simulink model "koen_observer_pll_model_annotated"  (R2024b)
settings: Solver=FixedStepDiscrete  StartTime=0.0  StopTime=0.05  FixedStep=6.25e-05  RelTol=1e-3
PreLoadFcn:
  | FOC_TS_SEC=6.25e-05; FOC_RS_OHM=0.53; FOC_LS_H=0.0006; FOC_FLUX_WB=0.0078; FOC_FLUX_LIMIT_RATIO=1.5; FOC_OBS_PLL_KP=180; FOC_OBS_PLL_KI=6000; FOC_OBS_PLL_INTEGRAL_LIMIT=700; FOC_OBS_SPEED_LIMIT_RAD_S=1200; FOC_OBS_SPEED_FILTER_ALPHA=0.2; FOC_OBS_THETA_COMP_RAD=2.7239; FOC_TWO_PI=6.283185307179586;
settings Model: Creator=10095  LastModifiedBy=10095

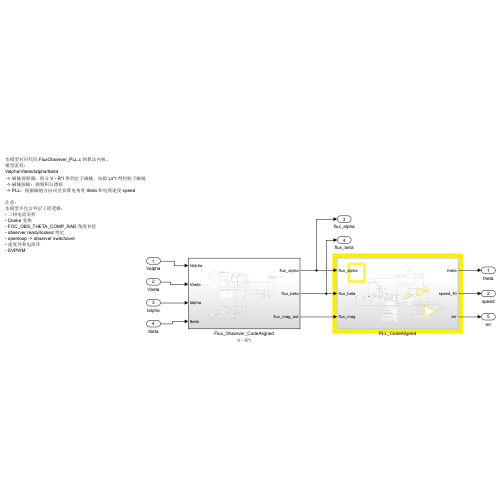
[thumbnail: Simulink's stored preview of the top-level diagram]
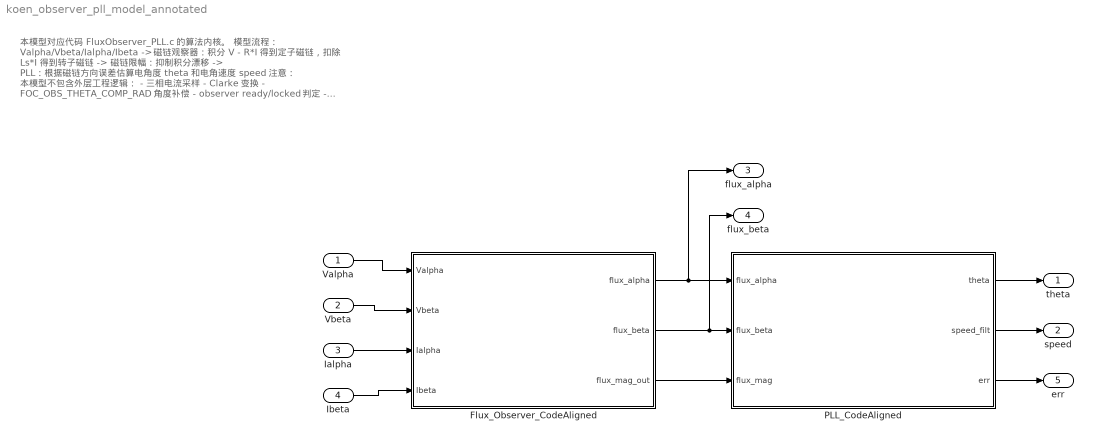
== system koen_observer_pll_model_annotated ==
  note: 本模型对应代码 FluxObserver_PLL.c 的算法内核。
      | 模型流程：
      | Valpha/Vbeta/Ialpha/Ibeta
      |  -> 磁链观察器：积分 V - R*I 得到定子磁链，扣除 Ls*I 得到转子磁链
      |  -> 磁链限幅：抑制积分漂移
      |  -> PLL：根据磁链方向误差估算电角度 theta 和电角速度 speed
      |
      | 注意：
      | 本模型不包含外层工程逻辑：
      | - 三相电流采样
      | - Clarke 变换
      | - FOC_OBS_THETA_COMP_RAD 角度补偿
      | - observer ready/locked 判定
      | - openloop -> observer switchover
      | - 速度环和电流环
      | - SVPWM
  Valpha : Inport
  Vbeta : Inport  Port=2
  Ialpha : Inport  Port=3
  Ibeta : Inport  Port=4
  Flux_Observer_CodeAligned : Subsystem  Description=|
      | Flux_Observer_CodeAligned：按 FluxObserver_PLL.c 更新定子磁链、扣除 Ls*i，并加入磁链幅值限幅。
      | 
      | 【代码对齐补充注释】
      | 定子磁链变化率计算模块。\n根据电机电压方程：psi_s_alpha_dot = Valpha - Rs*Ialpha。\nbeta 轴同理：psi_s_beta_dot = Vbeta - Rs*Ibeta。\n对应 FluxObserver_PLL.c 中 Ts * (ualpha - Rs*ialpha) 里的括号部分。
      settings: AttributesFormatString=V - R*I
  PLL_CodeAligned : Subsystem  Description=PLL_CodeAligned：按 FluxObserver_PLL.c 计算归一化相位误差、积分限幅、速度限幅、速度滤波和 theta wrap。
  theta : Outport
  speed : Outport  Port=2
  flux_alpha : Outport  Port=3
  flux_beta : Outport  Port=4
  err : Outport  Port=5
  wires:
  Valpha/1 -> Flux_Observer_CodeAligned/1(Valpha)
  Ialpha/1 -> Flux_Observer_CodeAligned/3(Ialpha)
  Vbeta/1 -> Flux_Observer_CodeAligned/2(Vbeta)
  Ibeta/1 -> Flux_Observer_CodeAligned/4(Ibeta)
  PLL_CodeAligned/1(theta) -> theta/1
  Flux_Observer_CodeAligned/3(flux_mag_out) -> PLL_CodeAligned/3(flux_mag)
  Flux_Observer_CodeAligned/2(flux_beta) -> PLL_CodeAligned/2(flux_beta), flux_beta/1
  PLL_CodeAligned/3(err) -> err/1
  Flux_Observer_CodeAligned/1(flux_alpha) -> flux_alpha/1, PLL_CodeAligned/1(flux_alpha)
  PLL_CodeAligned/2(speed_filt) -> speed/1

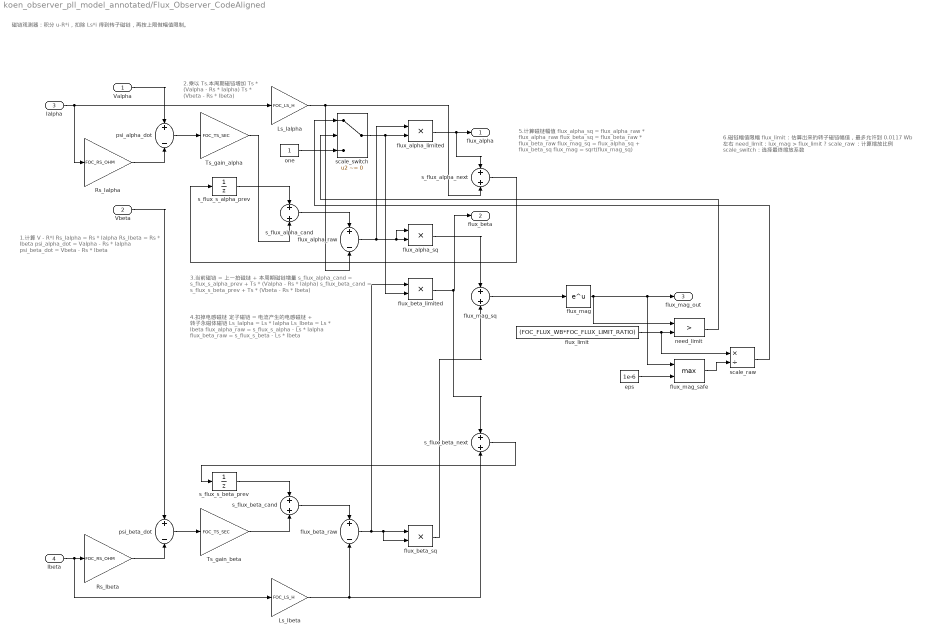
== system koen_observer_pll_model_annotated/Flux_Observer_CodeAligned ==
  note: 6.磁链幅值限幅
      | flux_limit：估算出来的转子磁链幅值，最多允许到 0.0117 Wb 左右
      | need_limit：lux_mag > flux_limit ?
      | scale_raw：计算缩放比例
      | scale_switch：选择最终缩放系数
  note: 5.计算磁链幅值
      | flux_alpha_sq = flux_alpha_raw * flux_alpha_raw
      | flux_beta_sq  = flux_beta_raw  * flux_beta_raw
      | flux_mag_sq   = flux_alpha_sq + flux_beta_sq
      | flux_mag      = sqrt(flux_mag_sq)
  note: 4.扣掉电感磁链
      | 定子磁链 = 电流产生的电感磁链 + 转子永磁体磁链
      | Ls_Ialpha = Ls * Ialpha
      | Ls_Ibeta  = Ls * Ibeta
      |
      | flux_alpha_raw = s_flux_s_alpha - Ls * Ialpha
      | flux_beta_raw  = s_flux_s_beta  - Ls * Ibeta
  note: 3.当前磁链 = 上一拍磁链 + 本周期磁链增量
      | s_flux_alpha_cand = s_flux_s_alpha_prev + Ts * (Valpha - Rs * Ialpha)
      | s_flux_beta_cand = s_flux_s_beta_prev + Ts * (Vbeta - Rs * Ibeta)
  note: 2.乘以 Ts.本周期磁链增加
      | Ts * (Valpha - Rs * Ialpha)
      | Ts * (Vbeta - Rs * Ibeta)
  note: 1.计算 V - R*I
      | Rs_Ialpha = Rs * Ialpha
      | Rs_Ibeta = Rs * Ibeta
      |
      | psi_alpha_dot = Valpha - Rs * Ialpha
      | psi_beta_dot = Vbeta - Rs * Ibeta
  note: 磁链观测器：积分 u-R*i，扣除 Ls*i 得到转子磁链，再按上限做幅值限制。
  Valpha : Inport  Description=|
      | 【代码对齐补充注释】
      | 输入端口：控制器输出的 alpha/beta 电压。\nValpha/Vbeta 对应代码 FluxObserver_PLL_t 中的 Valpha_I、Vbeta_I。\n这些电压是磁链积分的输入，来自电流环最终输出的 alpha/beta 电压。
      settings: AttributesFormatString=V - R*I
  Vbeta : Inport  Description=|  Port=2
      | 【代码对齐补充注释】
      | 输入端口：控制器输出的 alpha/beta 电压。\nValpha/Vbeta 对应代码 FluxObserver_PLL_t 中的 Valpha_I、Vbeta_I。\n这些电压是磁链积分的输入，来自电流环最终输出的 alpha/beta 电压。
      settings: AttributesFormatString=V - R*I
  Ialpha : Inport  Description=|  Port=3
      | 【代码对齐补充注释】
      | 输入端口：三相电流经过 Clarke 变换后的 alpha/beta 电流。\nIalpha/Ibeta 对应代码 FluxObserver_PLL_t 中的 Ialpha_I、Ibeta_I。\n这些电流用于计算 Rs*I 压降和 Ls*I 电感磁链。
      settings: AttributesFormatString=V - R*I
  Ibeta : Inport  Description=|  Port=4
      | 【代码对齐补充注释】
      | 输入端口：三相电流经过 Clarke 变换后的 alpha/beta 电流。\nIalpha/Ibeta 对应代码 FluxObserver_PLL_t 中的 Ialpha_I、Ibeta_I。\n这些电流用于计算 Rs*I 压降和 Ls*I 电感磁链。
      settings: AttributesFormatString=V - R*I
  Ls_Ialpha : Gain  Description=|  Gain=FOC_LS_H
      | 【代码对齐补充注释】
      | 输入端口：三相电流经过 Clarke 变换后的 alpha/beta 电流。\nIalpha/Ibeta 对应代码 FluxObserver_PLL_t 中的 Ialpha_I、Ibeta_I。\n这些电流用于计算 Rs*I 压降和 Ls*I 电感磁链。
      settings: AttributesFormatString=Ls * I
  Ls_Ibeta : Gain  Description=|  Gain=FOC_LS_H
      | 【代码对齐补充注释】
      | 输入端口：三相电流经过 Clarke 变换后的 alpha/beta 电流。\nIalpha/Ibeta 对应代码 FluxObserver_PLL_t 中的 Ialpha_I、Ibeta_I。\n这些电流用于计算 Rs*I 压降和 Ls*I 电感磁链。
      settings: AttributesFormatString=Ls * I
  Rs_Ialpha : Gain  Description=|  Gain=FOC_RS_OHM
      | 【代码对齐补充注释】
      | 输入端口：三相电流经过 Clarke 变换后的 alpha/beta 电流。\nIalpha/Ibeta 对应代码 FluxObserver_PLL_t 中的 Ialpha_I、Ibeta_I。\n这些电流用于计算 Rs*I 压降和 Ls*I 电感磁链。
      settings: AttributesFormatString=V - R*I
  Rs_Ibeta : Gain  Description=|  Gain=FOC_RS_OHM
      | 【代码对齐补充注释】
      | 输入端口：三相电流经过 Clarke 变换后的 alpha/beta 电流。\nIalpha/Ibeta 对应代码 FluxObserver_PLL_t 中的 Ialpha_I、Ibeta_I。\n这些电流用于计算 Rs*I 压降和 Ls*I 电感磁链。
      settings: AttributesFormatString=V - R*I
  Ts_gain_alpha : Gain  Description=|  Gain=FOC_TS_SEC
      | 【代码对齐补充注释】
      | 定子磁链变化率计算模块。\n根据电机电压方程：psi_s_alpha_dot = Valpha - Rs*Ialpha。\nbeta 轴同理：psi_s_beta_dot = Vbeta - Rs*Ibeta。\n对应 FluxObserver_PLL.c 中 Ts * (ualpha - Rs*ialpha) 里的括号部分。
      settings: AttributesFormatString=Ts * ψdot
  Ts_gain_beta : Gain  Description=|  Gain=FOC_TS_SEC
      | 【代码对齐补充注释】
      | 定子磁链变化率计算模块。\n根据电机电压方程：psi_s_alpha_dot = Valpha - Rs*Ialpha。\nbeta 轴同理：psi_s_beta_dot = Vbeta - Rs*Ibeta。\n对应 FluxObserver_PLL.c 中 Ts * (ualpha - Rs*ialpha) 里的括号部分。
      settings: AttributesFormatString=Ts * ψdot
  eps : Constant  Description=|  Value=1e-6
      | 【代码对齐补充注释】
      | 定子磁链变化率计算模块。\n根据电机电压方程：psi_s_alpha_dot = Valpha - Rs*Ialpha。\nbeta 轴同理：psi_s_beta_dot = Vbeta - Rs*Ibeta。\n对应 FluxObserver_PLL.c 中 Ts * (ualpha - Rs*ialpha) 里的括号部分。
      settings: AttributesFormatString=V - R*I
  flux_alpha_limited : Product  Description=|
      | 【代码对齐补充注释】
      | 定子磁链变化率计算模块。\n根据电机电压方程：psi_s_alpha_dot = Valpha - Rs*Ialpha。\nbeta 轴同理：psi_s_beta_dot = Vbeta - Rs*Ibeta。\n对应 FluxObserver_PLL.c 中 Ts * (ualpha - Rs*ialpha) 里的括号部分。
      settings: AttributesFormatString=limit |ψr|
  flux_alpha_raw : Sum  Description=|  Inputs=+-
      | 【代码对齐补充注释】
      | 定子磁链变化率计算模块。\n根据电机电压方程：psi_s_alpha_dot = Valpha - Rs*Ialpha。\nbeta 轴同理：psi_s_beta_dot = Vbeta - Rs*Ibeta。\n对应 FluxObserver_PLL.c 中 Ts * (ualpha - Rs*ialpha) 里的括号部分。
      settings: AttributesFormatString=ψr = ψs - LsI
  flux_alpha_sq : Product  Description=|
      | 【代码对齐补充注释】
      | 定子磁链变化率计算模块。\n根据电机电压方程：psi_s_alpha_dot = Valpha - Rs*Ialpha。\nbeta 轴同理：psi_s_beta_dot = Vbeta - Rs*Ibeta。\n对应 FluxObserver_PLL.c 中 Ts * (ualpha - Rs*ialpha) 里的括号部分。
      settings: AttributesFormatString=V - R*I
  flux_beta_limited : Product  Description=|
      | 【代码对齐补充注释】
      | 定子磁链变化率计算模块。\n根据电机电压方程：psi_s_alpha_dot = Valpha - Rs*Ialpha。\nbeta 轴同理：psi_s_beta_dot = Vbeta - Rs*Ibeta。\n对应 FluxObserver_PLL.c 中 Ts * (ualpha - Rs*ialpha) 里的括号部分。
      settings: AttributesFormatString=limit |ψr|
  flux_beta_raw : Sum  Description=|  Inputs=+-
      | 【代码对齐补充注释】
      | 定子磁链变化率计算模块。\n根据电机电压方程：psi_s_alpha_dot = Valpha - Rs*Ialpha。\nbeta 轴同理：psi_s_beta_dot = Vbeta - Rs*Ibeta。\n对应 FluxObserver_PLL.c 中 Ts * (ualpha - Rs*ialpha) 里的括号部分。
      settings: AttributesFormatString=ψr = ψs - LsI
  flux_beta_sq : Product  Description=|
      | 【代码对齐补充注释】
      | 定子磁链变化率计算模块。\n根据电机电压方程：psi_s_alpha_dot = Valpha - Rs*Ialpha。\nbeta 轴同理：psi_s_beta_dot = Vbeta - Rs*Ibeta。\n对应 FluxObserver_PLL.c 中 Ts * (ualpha - Rs*ialpha) 里的括号部分。
      settings: AttributesFormatString=V - R*I
  flux_limit : Constant  Description=|  Value=(FOC_FLUX_WB*FOC_FLUX_LIMIT_RATIO)
      | 【代码对齐补充注释】
      | 定子磁链变化率计算模块。\n根据电机电压方程：psi_s_alpha_dot = Valpha - Rs*Ialpha。\nbeta 轴同理：psi_s_beta_dot = Vbeta - Rs*Ibeta。\n对应 FluxObserver_PLL.c 中 Ts * (ualpha - Rs*ialpha) 里的括号部分。
      settings: AttributesFormatString=limit |ψr|
  flux_mag : Math  Description=|
      | 【代码对齐补充注释】
      | 定子磁链变化率计算模块。\n根据电机电压方程：psi_s_alpha_dot = Valpha - Rs*Ialpha。\nbeta 轴同理：psi_s_beta_dot = Vbeta - Rs*Ibeta。\n对应 FluxObserver_PLL.c 中 Ts * (ualpha - Rs*ialpha) 里的括号部分。
      settings: AttributesFormatString=|ψr|
  flux_mag_safe : MinMax  Description=|  Function=max  Inputs=2
      | 【代码对齐补充注释】
      | 定子磁链变化率计算模块。\n根据电机电压方程：psi_s_alpha_dot = Valpha - Rs*Ialpha。\nbeta 轴同理：psi_s_beta_dot = Vbeta - Rs*Ibeta。\n对应 FluxObserver_PLL.c 中 Ts * (ualpha - Rs*ialpha) 里的括号部分。
      settings: AttributesFormatString=|ψr|
  flux_mag_sq : Sum  Description=|
      | 【代码对齐补充注释】
      | 定子磁链变化率计算模块。\n根据电机电压方程：psi_s_alpha_dot = Valpha - Rs*Ialpha。\nbeta 轴同理：psi_s_beta_dot = Vbeta - Rs*Ibeta。\n对应 FluxObserver_PLL.c 中 Ts * (ualpha - Rs*ialpha) 里的括号部分。
      settings: AttributesFormatString=|ψr|
  need_limit : RelationalOperator  Description=|  Operator=>  OutDataTypeStr=boolean  RndMeth=Simplest  InputSameDT=off
      | 【代码对齐补充注释】
      | 定子磁链变化率计算模块。\n根据电机电压方程：psi_s_alpha_dot = Valpha - Rs*Ialpha。\nbeta 轴同理：psi_s_beta_dot = Vbeta - Rs*Ibeta。\n对应 FluxObserver_PLL.c 中 Ts * (ualpha - Rs*ialpha) 里的括号部分。
      settings: AttributesFormatString=limit |ψr|
  one : Constant  Description=|
      | 【代码对齐补充注释】
      | 定子磁链变化率计算模块。\n根据电机电压方程：psi_s_alpha_dot = Valpha - Rs*Ialpha。\nbeta 轴同理：psi_s_beta_dot = Vbeta - Rs*Ibeta。\n对应 FluxObserver_PLL.c 中 Ts * (ualpha - Rs*ialpha) 里的括号部分。
      settings: AttributesFormatString=V - R*I
  psi_alpha_dot : Sum  Description=|  Inputs=+-
      | 【代码对齐补充注释】
      | 定子磁链变化率计算模块。\n根据电机电压方程：psi_s_alpha_dot = Valpha - Rs*Ialpha。\nbeta 轴同理：psi_s_beta_dot = Vbeta - Rs*Ibeta。\n对应 FluxObserver_PLL.c 中 Ts * (ualpha - Rs*ialpha) 里的括号部分。
      settings: AttributesFormatString=V - R*I
  psi_beta_dot : Sum  Description=|  Inputs=+-
      | 【代码对齐补充注释】
      | 定子磁链变化率计算模块。\n根据电机电压方程：psi_s_alpha_dot = Valpha - Rs*Ialpha。\nbeta 轴同理：psi_s_beta_dot = Vbeta - Rs*Ibeta。\n对应 FluxObserver_PLL.c 中 Ts * (ualpha - Rs*ialpha) 里的括号部分。
      settings: AttributesFormatString=V - R*I
  s_flux_alpha_cand : Sum  Description=|
      | 【代码对齐补充注释】
      | 定子磁链变化率计算模块。\n根据电机电压方程：psi_s_alpha_dot = Valpha - Rs*Ialpha。\nbeta 轴同理：psi_s_beta_dot = Vbeta - Rs*Ibeta。\n对应 FluxObserver_PLL.c 中 Ts * (ualpha - Rs*ialpha) 里的括号部分。
      settings: AttributesFormatString=V - R*I
  s_flux_alpha_next : Sum  Description=|
      | 【代码对齐补充注释】
      | 定子磁链变化率计算模块。\n根据电机电压方程：psi_s_alpha_dot = Valpha - Rs*Ialpha。\nbeta 轴同理：psi_s_beta_dot = Vbeta - Rs*Ibeta。\n对应 FluxObserver_PLL.c 中 Ts * (ualpha - Rs*ialpha) 里的括号部分。
      settings: AttributesFormatString=V - R*I
  s_flux_beta_cand : Sum  Description=|
      | 【代码对齐补充注释】
      | 定子磁链变化率计算模块。\n根据电机电压方程：psi_s_alpha_dot = Valpha - Rs*Ialpha。\nbeta 轴同理：psi_s_beta_dot = Vbeta - Rs*Ibeta。\n对应 FluxObserver_PLL.c 中 Ts * (ualpha - Rs*ialpha) 里的括号部分。
      settings: AttributesFormatString=V - R*I
  s_flux_beta_next : Sum  Description=|
      | 【代码对齐补充注释】
      | 定子磁链变化率计算模块。\n根据电机电压方程：psi_s_alpha_dot = Valpha - Rs*Ialpha。\nbeta 轴同理：psi_s_beta_dot = Vbeta - Rs*Ibeta。\n对应 FluxObserver_PLL.c 中 Ts * (ualpha - Rs*ialpha) 里的括号部分。
      settings: AttributesFormatString=V - R*I
  s_flux_s_alpha_prev : UnitDelay  Description=|  InitialCondition=FOC_FLUX_WB  SampleTime=FOC_TS_SEC  HasFrameUpgradeWarning=on
      | 【代码对齐补充注释】
      | 定子磁链变化率计算模块。\n根据电机电压方程：psi_s_alpha_dot = Valpha - Rs*Ialpha。\nbeta 轴同理：psi_s_beta_dot = Vbeta - Rs*Ibeta。\n对应 FluxObserver_PLL.c 中 Ts * (ualpha - Rs*ialpha) 里的括号部分。
      settings: AttributesFormatString=ψs
  s_flux_s_beta_prev : UnitDelay  Description=|  SampleTime=FOC_TS_SEC  HasFrameUpgradeWarning=on
      | 【代码对齐补充注释】
      | 定子磁链变化率计算模块。\n根据电机电压方程：psi_s_alpha_dot = Valpha - Rs*Ialpha。\nbeta 轴同理：psi_s_beta_dot = Vbeta - Rs*Ibeta。\n对应 FluxObserver_PLL.c 中 Ts * (ualpha - Rs*ialpha) 里的括号部分。
      settings: AttributesFormatString=ψs
  scale_raw : Product  Description=|  Inputs=*/
      | 【代码对齐补充注释】
      | 定子磁链变化率计算模块。\n根据电机电压方程：psi_s_alpha_dot = Valpha - Rs*Ialpha。\nbeta 轴同理：psi_s_beta_dot = Vbeta - Rs*Ibeta。\n对应 FluxObserver_PLL.c 中 Ts * (ualpha - Rs*ialpha) 里的括号部分。
      settings: AttributesFormatString=limit |ψr|
  scale_switch : Switch  Description=|  Criteria=u2 ~= 0  Threshold=0.5  SaturateOnIntegerOverflow=off  InputSameDT=off
      | 【代码对齐补充注释】
      | 定子磁链变化率计算模块。\n根据电机电压方程：psi_s_alpha_dot = Valpha - Rs*Ialpha。\nbeta 轴同理：psi_s_beta_dot = Vbeta - Rs*Ibeta。\n对应 FluxObserver_PLL.c 中 Ts * (ualpha - Rs*ialpha) 里的括号部分。
      settings: AttributesFormatString=limit |ψr|
  flux_alpha : Outport  Description=|
      | 【代码对齐补充注释】
      | 定子磁链变化率计算模块。\n根据电机电压方程：psi_s_alpha_dot = Valpha - Rs*Ialpha。\nbeta 轴同理：psi_s_beta_dot = Vbeta - Rs*Ibeta。\n对应 FluxObserver_PLL.c 中 Ts * (ualpha - Rs*ialpha) 里的括号部分。
      settings: AttributesFormatString=V - R*I
  flux_beta : Outport  Description=|  Port=2
      | 【代码对齐补充注释】
      | 定子磁链变化率计算模块。\n根据电机电压方程：psi_s_alpha_dot = Valpha - Rs*Ialpha。\nbeta 轴同理：psi_s_beta_dot = Vbeta - Rs*Ibeta。\n对应 FluxObserver_PLL.c 中 Ts * (ualpha - Rs*ialpha) 里的括号部分。
      settings: AttributesFormatString=V - R*I
  flux_mag_out : Outport  Description=|  Port=3
      | 【代码对齐补充注释】
      | 定子磁链变化率计算模块。\n根据电机电压方程：psi_s_alpha_dot = Valpha - Rs*Ialpha。\nbeta 轴同理：psi_s_beta_dot = Vbeta - Rs*Ibeta。\n对应 FluxObserver_PLL.c 中 Ts * (ualpha - Rs*ialpha) 里的括号部分。
      settings: AttributesFormatString=|ψr|
  wires:
  Vbeta/1 -> psi_beta_dot/1
  Ibeta/1 -> Ls_Ibeta/1, Rs_Ibeta/1
  Ialpha/1 -> Ls_Ialpha/1, Rs_Ialpha/1
  s_flux_s_alpha_prev/1 -> s_flux_alpha_cand/1
  Valpha/1 -> psi_alpha_dot/1
  Rs_Ialpha/1 -> psi_alpha_dot/2
  Rs_Ibeta/1 -> psi_beta_dot/2
  psi_alpha_dot/1 -> Ts_gain_alpha/1
  psi_beta_dot/1 -> Ts_gain_beta/1
  Ts_gain_alpha/1 -> s_flux_alpha_cand/2
  flux_limit/1 -> need_limit/2, scale_raw/1
  flux_mag/1 -> flux_mag_safe/1, flux_mag_out/1, need_limit/1
  s_flux_s_beta_prev/1 -> s_flux_beta_cand/1
  Ts_gain_beta/1 -> s_flux_beta_cand/2
  Ls_Ialpha/1 -> flux_alpha_raw/2, s_flux_alpha_next/2
  one/1 -> scale_switch/3
  s_flux_alpha_cand/1 -> flux_alpha_raw/1
  s_flux_alpha_next/1 -> s_flux_s_alpha_prev/1
  flux_alpha_limited/1 -> s_flux_alpha_next/1, flux_alpha/1
  s_flux_beta_cand/1 -> flux_beta_raw/1
  s_flux_beta_next/1 -> s_flux_s_beta_prev/1
  flux_beta_limited/1 -> s_flux_beta_next/1, flux_beta/1
  Ls_Ibeta/1 -> s_flux_beta_next/2, flux_beta_raw/2
  scale_raw/1 -> scale_switch/1
  scale_switch/1 -> flux_alpha_limited/2, flux_beta_limited/2
  flux_alpha_raw/1 -> flux_alpha_sq/1, flux_alpha_sq/2, flux_alpha_limited/1
  flux_beta_raw/1 -> flux_beta_sq/2, flux_beta_sq/1, flux_beta_limited/1
  flux_beta_sq/1 -> flux_mag_sq/2
  flux_alpha_sq/1 -> flux_mag_sq/1
  flux_mag_sq/1 -> flux_mag/1
  eps/1 -> flux_mag_safe/2
  need_limit/1 -> scale_switch/2
  flux_mag_safe/1 -> scale_raw/2

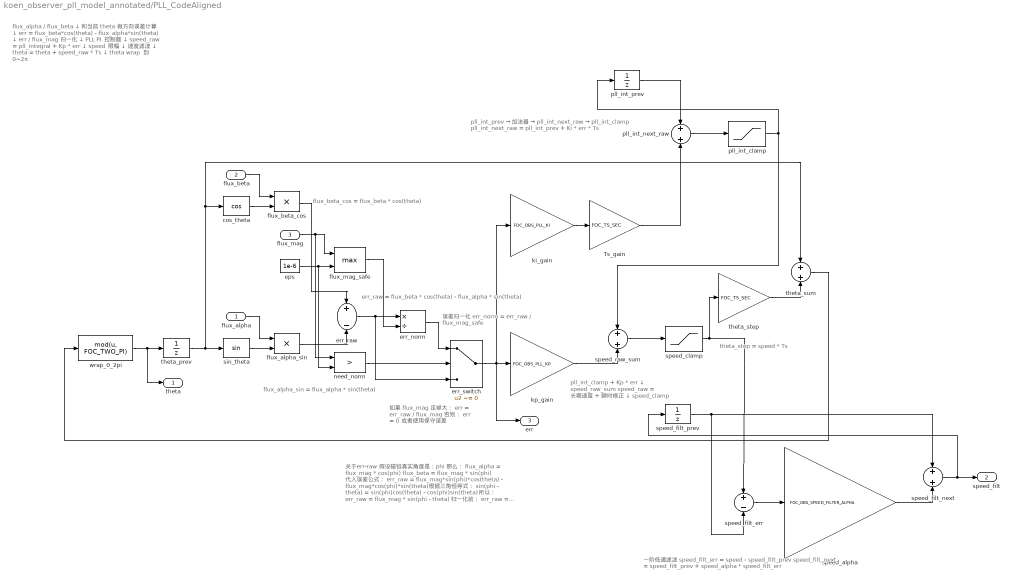
== system koen_observer_pll_model_annotated/PLL_CodeAligned ==
  note: 一阶低通滤波
      | speed_filt_err = speed - speed_filt_prev
      | speed_filt_next = speed_filt_prev + speed_alpha * speed_filt_err
  note: theta_step = speed * Ts
  note: pll_int_clamp
      | +
      | Kp * err
      | ↓
      | speed_raw_sum
      | speed_raw = 长期速度 + 瞬时修正
      | ↓
      | speed_clamp
  note: pll_int_prev → 加法器 → pll_int_next_raw → pll_int_clamp
      | pll_int_next_raw = pll_int_prev + Ki * err * Ts
  note: 如果 flux_mag 足够大：
      |     err = err_raw / flux_mag
      | 否则：
      |     err = 0 或者使用保守误差
  note: 误差归一化
      | err_norm = err_raw / flux_mag_safe
  note: 关于err-raw
      | 假设磁链真实角度是：phi
      | 那么：
      | flux_alpha = flux_mag * cos(phi)
      | flux_beta = flux_mag * sin(phi)
      | 代入误差公式：
      | err_raw = flux_mag*sin(phi)*cos(theta)
      | - flux_mag*cos(phi)*sin(theta)
      | 根据三角恒等式：
      | sin(phi - theta) = sin(phi)cos(theta) - cos(phi)sin(theta)
      | 所以：
      | err_raw = flux_mag * sin(phi - theta)
      | 归一化前：
      | err_raw = 磁链幅值 × sin(真实角度 - PLL估计角度)
      | 所以：
      | err_raw > 0 PLL 角度落后了，需要加速追上
      | err_raw < 0 PLL 角度超前了，需要减速回来
      | err_raw = 0 PLL 角度和磁链方向对齐
  note: err_raw = flux_beta * cos(theta) - flux_alpha * sin(theta)
  note: flux_alpha_sin = flux_alpha * sin(theta)
  note: flux_beta_cos = flux_beta * cos(theta)
  note: flux_alpha / flux_beta
      |         ↓
      | 和当前 theta 做方向误差计算
      |         ↓
      | err = flux_beta*cos(theta) - flux_alpha*sin(theta)
      |         ↓
      | err / flux_mag 归一化
      |         ↓
      | PLL PI 控制器
      |         ↓
      | speed_raw = pll_integral + Kp * err
      |         ↓
      | speed 限幅
      |         ↓
      | 速度滤波
      |         ↓
      | theta = theta + speed_raw * Ts
      |         ↓
      | theta wrap 到 0~2π
  flux_alpha : Inport  Description=|
      | 【代码对齐补充注释】
      | PLL 输入：来自磁链观察器的转子磁链矢量和幅值。\nPLL 用 flux_alpha/flux_beta 追踪磁链方向，并用 flux_mag 做误差归一化。
      settings: AttributesFormatString=LPF speed
  flux_beta : Inport  Description=|  Port=2
      | 【代码对齐补充注释】
      | PLL 输入：来自磁链观察器的转子磁链矢量和幅值。\nPLL 用 flux_alpha/flux_beta 追踪磁链方向，并用 flux_mag 做误差归一化。
      settings: AttributesFormatString=PLL 输入
  flux_mag : Inport  Description=|  Port=3
      | 【代码对齐补充注释】
      | PLL 输入：来自磁链观察器的转子磁链矢量和幅值。\nPLL 用 flux_alpha/flux_beta 追踪磁链方向，并用 flux_mag 做误差归一化。
      settings: AttributesFormatString=PLL 输入
  Ts_gain : Gain  Gain=FOC_TS_SEC
  cos_theta : Trigonometry  Description=|  Operator=cos
      | 【代码对齐补充注释】
      | 根据当前估计角度生成单位方向向量。\n[cos(theta), sin(theta)] 表示 PLL 当前认为的磁链方向。
      settings: AttributesFormatString=sin/cos θ
  eps : Constant  Description=|  Value=1e-6
      | 【代码对齐补充注释】
      | PLL 误差归一化模块。\n公式：err = err_raw / flux_mag。\n归一化后 err 近似等于角度误差。\n使用 eps 或安全幅值，防止 flux_mag 接近 0 时除零。
      settings: AttributesFormatString=err / |ψ|
  err_norm : Product  Description=|  Inputs=*/
      | 【代码对齐补充注释】
      | PLL 误差归一化模块。\n公式：err = err_raw / flux_mag。\n归一化后 err 近似等于角度误差。\n使用 eps 或安全幅值，防止 flux_mag 接近 0 时除零。
      settings: AttributesFormatString=Kp*err
  err_raw : Sum  Description=|  Inputs=+-
      | 【代码对齐补充注释】
      | PLL 正交误差计算模块。\n公式：err_raw = flux_beta*cos(theta) - flux_alpha*sin(theta)。\n等价于 flux_mag * sin(phi - theta)。\nerr_raw > 0 表示 PLL 落后，需要加速；err_raw < 0 表示 PLL 超前，需要减速；err_raw = 0 表示对准。
      settings: AttributesFormatString=Kp*err
  err_switch : Switch  Description=|  Criteria=u2 ~= 0  Threshold=0.5  SaturateOnIntegerOverflow=off  InputSameDT=off
      | 【代码对齐补充注释】
      | PLL 比例通道。\n公式：p_term = Kp * err。\n作用：快速修正瞬时角度误差。
      settings: AttributesFormatString=Kp*err
  flux_alpha_sin : Product  Description=|
      | 【代码对齐补充注释】
      | PLL 输入：来自磁链观察器的转子磁链矢量和幅值。\nPLL 用 flux_alpha/flux_beta 追踪磁链方向，并用 flux_mag 做误差归一化。
      settings: AttributesFormatString=LPF speed
  flux_beta_cos : Product  Description=|
      | 【代码对齐补充注释】
      | PLL 输入：来自磁链观察器的转子磁链矢量和幅值。\nPLL 用 flux_alpha/flux_beta 追踪磁链方向，并用 flux_mag 做误差归一化。
      settings: AttributesFormatString=sin/cos θ
  flux_mag_safe : MinMax  Description=|  Function=max  Inputs=2
      | 【代码对齐补充注释】
      | PLL 输入：来自磁链观察器的转子磁链矢量和幅值。\nPLL 用 flux_alpha/flux_beta 追踪磁链方向，并用 flux_mag 做误差归一化。
      settings: AttributesFormatString=err / |ψ|
  ki_gain : Gain  Description=|  Gain=FOC_OBS_PLL_KI
      | 【代码对齐补充注释】
      | PLL 积分通道增量。\n公式：pll_integral += Ki * err * Ts。\n作用：更新速度积分项，消除稳态角度误差。
      settings: AttributesFormatString=Ki*err*Ts
  kp_gain : Gain  Description=|  Gain=FOC_OBS_PLL_KP
      | 【代码对齐补充注释】
      | PLL 比例通道。\n公式：p_term = Kp * err。\n作用：快速修正瞬时角度误差。
      settings: AttributesFormatString=Kp*err
  need_norm : RelationalOperator  Operator=>  OutDataTypeStr=boolean  RndMeth=Simplest  InputSameDT=off
  pll_int_clamp : Saturate  UpperLimit=FOC_OBS_PLL_INTEGRAL_LIMIT  LowerLimit=-FOC_OBS_PLL_INTEGRAL_LIMIT
  pll_int_next_raw : Sum
  pll_int_prev : UnitDelay  SampleTime=FOC_TS_SEC  HasFrameUpgradeWarning=on
  sin_theta : Trigonometry  Description=|
      | 【代码对齐补充注释】
      | 根据当前估计角度生成单位方向向量。\n[cos(theta), sin(theta)] 表示 PLL 当前认为的磁链方向。
      settings: AttributesFormatString=sin/cos θ
  speed_alpha : Gain  Description=|  Gain=FOC_OBS_SPEED_FILTER_ALPHA
      | 【代码对齐补充注释】
      | 速度一阶低通滤波模块。\n公式：speed_filt = speed_filt_prev + alpha*(speed_raw - speed_filt_prev)。\n用于给外部速度环提供更平滑的速度反馈。
      settings: AttributesFormatString=LPF speed
  speed_clamp : Saturate  Description=|  UpperLimit=FOC_OBS_SPEED_LIMIT_RAD_S  LowerLimit=-FOC_OBS_SPEED_LIMIT_RAD_S
      | 【代码对齐补充注释】
      | observer 电角速度限幅模块。\n对应 FOC_OBS_SPEED_LIMIT_RAD_S。\n如果命中限幅，对应运行日志 speed_limit_hit / lim_s = 1。
      settings: AttributesFormatString=clamp speed
  speed_filt_err : Sum  Description=|  Inputs=+-
      | 【代码对齐补充注释】
      | PLL 比例通道。\n公式：p_term = Kp * err。\n作用：快速修正瞬时角度误差。
      settings: AttributesFormatString=Kp*err
  speed_filt_next : Sum
  speed_filt_prev : UnitDelay  SampleTime=FOC_TS_SEC  HasFrameUpgradeWarning=on
  speed_raw_sum : Sum  Description=|
      | 【代码对齐补充注释】
      | PLL 原始电角速度计算模块。\n公式：speed_raw = pll_integral + Kp*err。\n对应代码中的 s_speed_rad_s 限幅前后原始速度路径。
      settings: AttributesFormatString=speed_raw
  theta_prev : UnitDelay  Description=|  SampleTime=FOC_TS_SEC  HasFrameUpgradeWarning=on
      | 【代码对齐补充注释】
      | 上一拍 PLL 角度保存模块。\ntheta 是 PLL 当前估计的磁链方向角。\n对应代码中的 s_theta_rad 状态变量。
      settings: AttributesFormatString=theta z^-1
  theta_step : Gain  Description=|  Gain=FOC_TS_SEC
      | 【代码对齐补充注释】
      | 角度积分模块。\n用电角速度积分得到下一拍角度。\n公式：theta_next = theta_prev + speed_raw * Ts。
      settings: AttributesFormatString=θ += ωTs
  theta_sum : Sum  Description=|
      | 【代码对齐补充注释】
      | 角度积分模块。\n用电角速度积分得到下一拍角度。\n公式：theta_next = theta_prev + speed_raw * Ts。
      settings: AttributesFormatString=θ += ωTs
  wrap_0_2pi : Fcn  Description=|  Expr=mod(u, FOC_TWO_PI)
      | 【代码对齐补充注释】
      | 角度环绕模块。\n将 theta 限制到 [0, 2π)，防止角度无限增大。\n输出最终 PLL 电角度，对应代码中的 Etheta_O。
      settings: AttributesFormatString=wrap 0..2π
  theta : Outport
  speed_filt : Outport  Port=2
  err : Outport  Description=|  Port=3
      | 【代码对齐补充注释】
      | PLL 比例通道。\n公式：p_term = Kp * err。\n作用：快速修正瞬时角度误差。
      settings: AttributesFormatString=Kp*err
  wires:
  wrap_0_2pi/1 -> theta_prev/1, theta/1
  theta_prev/1 -> theta_sum/1, cos_theta/1, sin_theta/1
  flux_alpha/1 -> flux_alpha_sin/1
  flux_beta/1 -> flux_beta_cos/1
  err_raw/1 -> err_switch/3, err_norm/1
  flux_beta_cos/1 -> err_raw/1
  sin_theta/1 -> flux_alpha_sin/2
  flux_alpha_sin/1 -> err_raw/2
  cos_theta/1 -> flux_beta_cos/2
  flux_mag/1 -> need_norm/1, flux_mag_safe/1
  need_norm/1 -> err_switch/2
  eps/1 -> need_norm/2, flux_mag_safe/2
  flux_mag_safe/1 -> err_norm/2
  err_norm/1 -> err_switch/1
  err_switch/1 -> ki_gain/1, kp_gain/1, err/1
  ki_gain/1 -> Ts_gain/1
  kp_gain/1 -> speed_raw_sum/2
  pll_int_prev/1 -> pll_int_next_raw/1
  pll_int_clamp/1 -> pll_int_prev/1, speed_raw_sum/1
  Ts_gain/1 -> pll_int_next_raw/2
  speed_raw_sum/1 -> speed_clamp/1
  pll_int_next_raw/1 -> pll_int_clamp/1
  speed_clamp/1 -> speed_filt_err/1, theta_step/1
  speed_filt_prev/1 -> speed_filt_err/2, speed_filt_next/1
  theta_step/1 -> theta_sum/2
  speed_filt_err/1 -> speed_alpha/1
  theta_sum/1 -> wrap_0_2pi/1
  speed_alpha/1 -> speed_filt_next/2
  speed_filt_next/1 -> speed_filt/1, speed_filt_prev/1
